simulink model "lab3"  (R2018b)
settings: Solver=ode4  StartTime=0.0  StopTime=100  FixedStep=2^-5  RelTol=1e-3
libraries: simulink x2
settings Model: Creator=vandavv  LastModifiedBy=vandavv

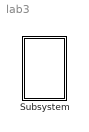
== system lab3 ==
  Subsystem : Subsystem  mask{g=9.81, l=2, m=2, k=5, r0=3, r1=1, f0=0.1, f1=0.1}

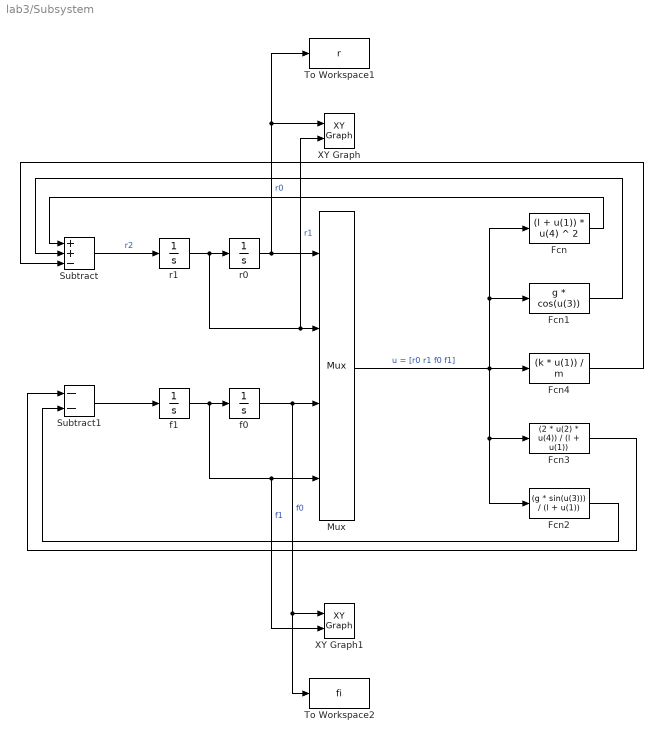
== system lab3/Subsystem ==
  Fcn : Fcn  Expr=(l + u(1)) * u(4) ^ 2
  Fcn1 : Fcn  Expr=g * cos(u(3))
  Fcn2 : Fcn  Expr=(g * sin(u(3))) / (l + u(1))
  Fcn3 : Fcn  Expr=(2 * u(2) * u(4)) / (l + u(1))
  Fcn4 : Fcn  Expr=(k * u(1)) / m
  Mux : Mux
  Subtract : Sum  Inputs=++-
  Subtract1 : Sum  Inputs=--
  To Workspace1 : ToWorkspace  VariableName=r  SampleTime=-1
  To Workspace2 : ToWorkspace  VariableName=fi  SampleTime=-1
  XY Graph : simulink/Sinks/XY Graph  xmin=2.5  xmax=5.5  ymin=-2  ymax=2  st=-1
  XY Graph1 : simulink/Sinks/XY Graph  xmin=-0.2  xmax=0.2  ymin=-0.2  ymax=0.2  st=-1
  f0 : Integrator  InitialCondition=f0
  f1 : Integrator  InitialCondition=f1
  r0 : Integrator  InitialCondition=r0
  r1 : Integrator  InitialCondition=r1
  wires:
  Fcn3/1 -> Subtract1/1
  Subtract/1 -> r1/1  "r2"
  Mux/1 -> Fcn2/1, Fcn3/1, Fcn4/1, Fcn1/1, Fcn/1  "u = [r0 r1 f0 f1]"
  Fcn/1 -> Subtract/1
  r0/1 -> To Workspace1/1, XY Graph/1, Mux/1  "r0"
  Subtract1/1 -> f1/1
  r1/1 -> XY Graph/2, Mux/2, r0/1  "r1"
  Fcn4/1 -> Subtract/3
  f0/1 -> To Workspace2/1, XY Graph1/1, Mux/3  "f0"
  Fcn1/1 -> Subtract/2
  f1/1 -> XY Graph1/2, Mux/4, f0/1  "f1"
  Fcn2/1 -> Subtract1/2
